simulink model "sampleModel1578"  (R2023a)
settings: Solver=VariableStepAuto  StartTime=0.0  StopTime=10.0  RelTol=1e-3
libraries: hdlsllib x5, simulink x4
settings Model: Creator=user1  LastModifiedBy=user1

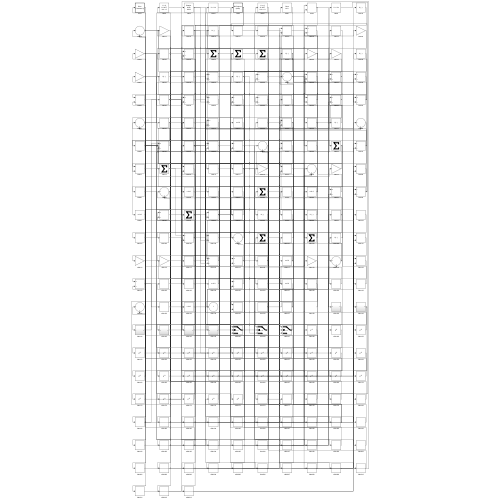
[thumbnail: Simulink's stored preview of the top-level diagram]
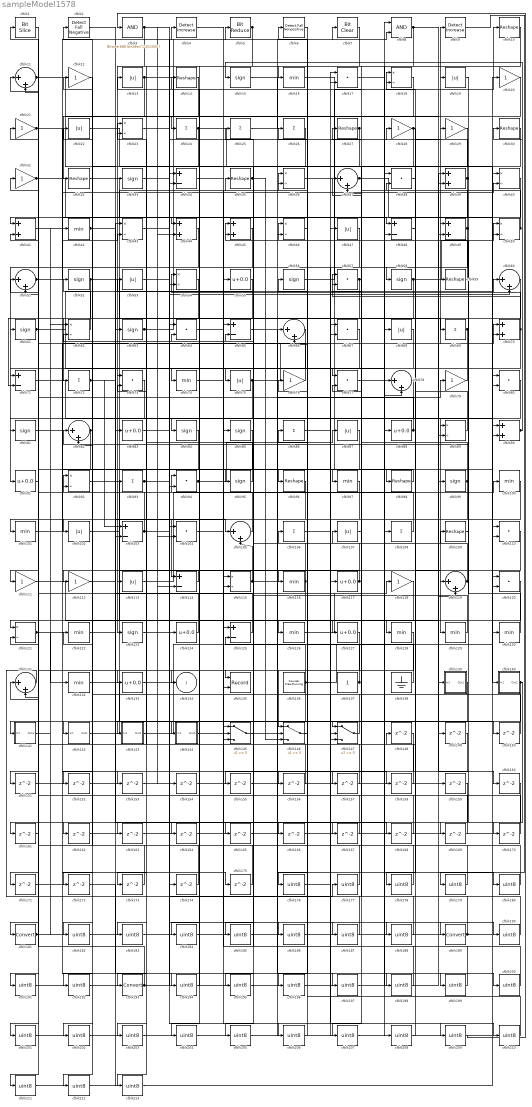
== system sampleModel1578 ==
  cfblk1 : hdlsllib/Logic and Bit Operations/Bit Slice  lidx=7  ridx=0
  cfblk{10,14,27,30,32,35,59,96,98,109} (10 alike) : Reshape
  cfblk{16,42,74,97,100..101,116,122,126,128..130,132} (13 alike) : MinMax
  cfblk{13,19,22,47,53,68,75,87,102,107,113} (11 alike) : Abs  SaturateOnIntegerOverflow=off
  cfblk{34,48,65,71,103,114,125} (7 alike) : Sum  Inputs=+-
  cfblk{17,38,57,64,67,73,77,80,94,104,110,120} (12 alike) : DotProduct  OutDataTypeStr=Inherit: Inherit via internal rule
  cfblk{11,37,51,60,66,78,82,105,119,131} (10 alike) : Sum  Inputs=|++
  cfblk{24..26,69,72,86,93,106,108} (9 alike) : Sum  Inputs=+
  cfblk{12,20..21,28..29,31,76,79,111..112,118} (11 alike) : Gain
  cfblk{18,23,36,40,43,46,50,54,62,89,92,115,121} (13 alike) : Product  Inputs=*/  RndMeth=Zero  SaturateOnIntegerOverflow=on
  cfblk{55,83,88,91,117,124,127,133} (8 alike) : Bias  Bias=0.0  SaturateOnIntegerOverflow=off
  cfblk{15,33,52,56,58,61,63,81,84..85,95,99,123} (13 alike) : Signum
  cfblk135 : Record  FileSettingsInternal="{\"entries\":[{\"content\":{\"excelSettings\":{\"content\":{},\"type\":\"Streamout.ExcelSettings\"}},\"type\":\"Streamout.FileSettingStorage\",\"uuid\":\"\"}],\"packageUris\":[\"http:\\/\\/schema.mathworks.com\\/mf0\\/streamout_blocks\\/R2020a\"],\"version\":\"1.0\"}"  Layout=[1 1]  SignalsInternal="{\"entries\":[{\"content\":{\"signals\":[{\"content\":{\"blockPath\":[],\"dimensions\":[1],\"domain\":\"\",\"lineColor\":\"#a2142f\",\"plots\":[1],\"port\":1,\"signalID\":1922,\"signalName\":\"XY Graph:1\"},\"type\":\"RecordBlkView.Signal\",\"uuid\":\"\"},{\"content\":{\"blockPath\":[],\"dimensions\":[1],\"domain\":\"\",\"lineColor\":\"#139fff\",\"plots\":[1],\"port\":2,\"signalID\":1925,\"signalName\":\"XY Graph:2\"},\"type\":\"RecordBlkView.Signal\",\"uuid\":\"\"}]},\"type\":\"RecordBlkView.InputSignals\",\"uuid\":\"\"}],\"packageUris\":[\"http:\\/\\/schema.mathworks.com\\/mf0\\/streamout_blocks\\/R2020a\"],\"version\":\"1.0\"}"  VisualizationBindings="{\"xyplotplugin\":{\"info\":[{\"series\":[{\"bindingParametersList\":[{\"parameter\":\"X-Axis\",\"signalID\":1922,\"signalName\":\"XY Graph:1\"},{\"parameter\":\"Y-Axis\",\"signalID\":1925,\"signalName\":\"XY Graph:2\"}],\"seriesID\":19021}],\"subplotID\":1}]}}"  CompatibilityTag=XY  st=-1
  cfblk136 : hdlsllib/Sources/Counter Free-Running  NumBits=16  tsamp=-1
  cfblk137 : Constant  SampleTime=-1
  cfblk138 : Ground
  cfblk139 : Subsystem
      settings: LibrarySourceBlock=|
      | hdlsllib/Ports &
      | Subsystems/Subsystem
  cfblk140 : Subsystem
      settings: LibrarySourceBlock=|
      | hdlsllib/Ports &
      | Subsystems/Subsystem
  cfblk141 : Subsystem
      settings: LibrarySourceBlock=|
      | hdlsllib/Ports &
      | Subsystems/Subsystem
  cfblk142 : Subsystem
      settings: LibrarySourceBlock=|
      | hdlsllib/Ports &
      | Subsystems/Subsystem
  cfblk143 : Subsystem
      settings: LibrarySourceBlock=|
      | hdlsllib/Ports &
      | Subsystems/Subsystem
  cfblk144 : Subsystem
      settings: LibrarySourceBlock=|
      | hdlsllib/Ports &
      | Subsystems/Subsystem
  cfblk145 : Switch  SaturateOnIntegerOverflow=off  InputSameDT=off
  cfblk146 : Switch  SaturateOnIntegerOverflow=off  InputSameDT=off
  cfblk147 : Switch  SaturateOnIntegerOverflow=off  InputSameDT=off
  cfblk{148..175} (28 alike) : Delay  SampleTime=1
  cfblk{176..180,182..188,190..192,194..213} (35 alike) : DataTypeConversion  OutDataTypeStr=uint8  SaturateOnIntegerOverflow=off  RndMeth=Floor
  cfblk181 : DataTypeConversion  SaturateOnIntegerOverflow=off  RndMeth=Floor
  cfblk189 : DataTypeConversion  SaturateOnIntegerOverflow=off  RndMeth=Floor
  cfblk193 : DataTypeConversion  SaturateOnIntegerOverflow=off  RndMeth=Floor
  cfblk2 : hdlsllib/Logic and Bit Operations/Detect Fall Negative  vinit=0  OutDataTypeStr=boolean
  cfblk3 : simulink/Logic and Bit Operations/Bitwise Operator  logicop=AND  UseBitMask=on  BitMask=bin2dec('11011001')  BitMaskRealWorld=Stored Integer
      settings: LibrarySourceBlock=|
      | hdlsllib/Logic and Bit
      | Operations/Bitwise
      | Operator
  cfblk{39,41,44..45,49,70,90} (7 alike) : Sum
  cfblk4 : simulink/Logic and Bit Operations/Detect Increase  vinit=0.0  OutDataTypeStr=boolean
      settings: LibrarySourceBlock=|
      | hdlsllib/Logic and Bit
      | Operations/Detect
      | Increase
  cfblk5 : hdlsllib/Logic and Bit Operations/Bit Reduce  mode=AND
  cfblk6 : hdlsllib/Logic and Bit Operations/Detect Fall Nonpositive  vinit=0  OutDataTypeStr=boolean
  cfblk7 : simulink/Logic and Bit Operations/Bit Clear  iBit=0
      settings: LibrarySourceBlock=|
      | hdlsllib/Logic and Bit
      | Operations/Bit Clear
  cfblk8 : Logic  AllPortsSameDT=off  OutDataTypeStr=boolean
  cfblk9 : simulink/Logic and Bit Operations/Detect Increase  vinit=0.0  OutDataTypeStr=boolean
      settings: LibrarySourceBlock=|
      | hdlsllib/Logic and Bit
      | Operations/Detect
      | Increase
  cfblk134 : Outport  VectorParamsAs1DForOutWhenUnconnected=off
  wires:
  cfblk141/1(Out1) -> cfblk42/1
  cfblk98/1 -> cfblk97/1
  cfblk63/1 -> cfblk5/1, cfblk7/1, cfblk104/2
  cfblk117/1 -> cfblk2/1, cfblk113/1
  cfblk44/1 -> cfblk91/1
  cfblk49/1 -> cfblk16/1, cfblk147/3
  cfblk108/1 -> cfblk94/1
  cfblk58/1 -> cfblk50/1, cfblk71/2
  cfblk90/1 -> cfblk15/1, cfblk30/1
  cfblk110/1 -> cfblk128/1
  cfblk59/1 -> cfblk45/1
  cfblk140/1(Out1) -> cfblk170/1, cfblk171/1
  cfblk43/1 -> cfblk124/1
  cfblk137/1 -> cfblk135/1, cfblk36/2
  cfblk56/1 -> cfblk28/1
  cfblk142/1(Out1) -> cfblk35/1
  cfblk129/1 -> cfblk45/2
  cfblk31/1 -> cfblk123/1, cfblk98/1
  cfblk32/1 -> cfblk48/1
  cfblk80/1 -> cfblk181/1
  cfblk132/1 -> cfblk147/1
  cfblk3/1 -> cfblk73/1, cfblk96/1, cfblk154/1
  cfblk18/1 -> cfblk24/1
  cfblk103/1 -> cfblk92/1, cfblk150/1
  cfblk130/1 -> cfblk82/1
  cfblk2/1 -> cfblk105/1
  cfblk40/1 -> cfblk116/1
  cfblk75/1 -> cfblk9/1, cfblk173/1, cfblk180/1
  cfblk55/1 -> cfblk61/1
  cfblk36/1 -> cfblk10/1
  cfblk69/1 -> cfblk82/2, cfblk169/1
  cfblk71/1 -> cfblk129/1
  cfblk52/1 -> cfblk121/1, cfblk94/2
  cfblk138/1 -> cfblk26/1
  cfblk14/1 -> cfblk193/1
  cfblk45/1 -> cfblk102/1
  cfblk37/1 -> cfblk140/1(In1), cfblk190/1
  cfblk144/1(Out1) -> cfblk100/1
  cfblk54/1 -> cfblk72/1
  cfblk62/1 -> cfblk52/1
  cfblk133/1 -> cfblk55/1
  cfblk143/1(Out1) -> cfblk20/1
  cfblk7/1 -> cfblk33/1
  cfblk16/1 -> cfblk130/1
  cfblk101/1 -> cfblk70/1
  cfblk61/1 -> cfblk19/1, cfblk104/1, cfblk93/1, cfblk108/1, cfblk175/1
  cfblk87/1 -> cfblk143/1(In1)
  cfblk48/1 -> cfblk18/1
  cfblk73/1 -> cfblk81/1
  cfblk124/1 -> cfblk21/1
  cfblk12/1 -> cfblk142/1(In1)
  cfblk8/1 -> cfblk48/2, cfblk160/1
  cfblk105/1 -> cfblk51/1
  cfblk82/1 -> cfblk111/1, cfblk152/1
  cfblk51/1 -> cfblk40/2, cfblk4/1
  cfblk24/1 -> cfblk68/1, cfblk192/1
  cfblk96/1 -> cfblk131/2
  cfblk29/1 -> cfblk34/2
  cfblk113/1 -> cfblk39/1
  cfblk109/1 -> cfblk49/1
  cfblk94/1 -> cfblk87/1, cfblk36/1
  cfblk72/1 -> cfblk77/1, cfblk103/1
  cfblk20/1 -> cfblk32/1
  cfblk57/1 -> cfblk166/1, cfblk167/1
  cfblk123/1 -> cfblk29/1
  cfblk22/1 -> cfblk50/2
  cfblk107/1 -> cfblk57/1
  cfblk76/1 -> cfblk11/1
  cfblk104/1 -> cfblk60/1
  cfblk122/1 -> cfblk118/1
  cfblk11/1 -> cfblk83/1, cfblk59/1
  cfblk84/1 -> cfblk101/1
  cfblk10/1 -> cfblk134/1
  cfblk111/1 -> cfblk139/1(In1)
  cfblk126/1 -> cfblk8/1
  cfblk5/1 -> cfblk163/1, cfblk203/1
  cfblk147/1 -> cfblk22/1
  cfblk35/1 -> cfblk146/3, cfblk185/1
  cfblk99/1 -> cfblk77/2, cfblk182/1
  cfblk88/1 -> cfblk84/1, cfblk51/2
  cfblk28/1 -> cfblk127/1, cfblk58/1
  cfblk102/1 -> cfblk126/1
  cfblk92/1 -> cfblk119/1
  cfblk34/1 -> cfblk115/1
  cfblk106/1 -> cfblk189/1
  cfblk79/1 -> cfblk74/1
  cfblk30/1 -> cfblk75/1
  cfblk121/1 -> cfblk132/1, cfblk200/1
  cfblk70/1 -> cfblk54/1, cfblk57/2, cfblk202/1
  cfblk50/1 -> cfblk13/1, cfblk44/1
  cfblk100/1 -> cfblk114/1
  cfblk125/1 -> cfblk23/1
  cfblk93/1 -> cfblk54/2, cfblk114/2
  cfblk41/1 -> cfblk43/2
  cfblk19/1 -> cfblk89/1
  cfblk95/1 -> cfblk73/2
  cfblk39/1 -> cfblk18/2, cfblk71/1
  cfblk83/1 -> cfblk145/3
  cfblk27/1 -> cfblk95/1, cfblk165/1
  cfblk13/1 -> cfblk125/1, cfblk44/2, cfblk162/1, cfblk213/1
  cfblk128/1 -> cfblk146/1
  cfblk114/1 -> cfblk112/1
  cfblk146/1 -> cfblk76/1
  cfblk127/1 -> cfblk141/1(In1)
  cfblk89/1 -> cfblk46/1
  cfblk21/1 -> cfblk46/2, cfblk194/1
  cfblk85/1 -> cfblk133/1
  cfblk17/1 -> cfblk90/2
  cfblk25/1 -> cfblk8/2
  cfblk116/1 -> cfblk53/1, cfblk155/1
  cfblk68/1 -> cfblk144/1(In1)
  cfblk115/1 -> cfblk79/1, cfblk105/2
  cfblk33/1 -> cfblk60/2
  cfblk1/1 -> cfblk41/1
  cfblk97/1 -> cfblk135/2
  cfblk119/1 -> cfblk109/1, cfblk37/2
  cfblk136/1 -> cfblk89/2, cfblk146/2, cfblk25/1
  cfblk42/1 -> cfblk69/1, cfblk147/2, cfblk168/1
  cfblk150/1 -> cfblk34/1
  cfblk139/1(Out1) -> cfblk151/1
  cfblk151/1 -> cfblk115/2
  cfblk152/1 -> cfblk92/2
  cfblk81/1 -> cfblk153/1
  cfblk154/1 -> cfblk119/2
  cfblk155/1 -> cfblk125/2
  cfblk53/1 -> cfblk156/1
  cfblk156/1 -> cfblk23/2
  cfblk4/1 -> cfblk157/1
  cfblk157/1 -> cfblk131/1
  cfblk112/1 -> cfblk158/1
  cfblk158/1 -> cfblk43/1
  cfblk91/1 -> cfblk161/1
  cfblk161/1 -> cfblk121/2
  cfblk162/1 -> cfblk70/2
  cfblk163/1 -> cfblk145/2
  cfblk60/1 -> cfblk164/1
  cfblk164/1 -> cfblk49/2
  cfblk165/1 -> cfblk17/2
  cfblk166/1 -> cfblk90/1
  cfblk167/1 -> cfblk11/2
  cfblk168/1 -> cfblk41/2
  cfblk169/1 -> cfblk37/1
  cfblk170/1 -> cfblk145/1
  cfblk171/1 -> cfblk103/2
  cfblk118/1 -> cfblk172/1
  cfblk173/1 -> cfblk62/2
  cfblk174/1 -> cfblk1/1
  cfblk175/1 -> cfblk12/1
  cfblk6/1 -> cfblk176/1
  cfblk176/1 -> cfblk117/1
  cfblk131/1 -> cfblk177/1
  cfblk177/1 -> cfblk6/1
  cfblk38/1 -> cfblk178/1
  cfblk178/1 -> cfblk122/1
  cfblk9/1 -> cfblk179/1
  cfblk179/1 -> cfblk38/1
  cfblk180/1 -> cfblk38/2
  cfblk181/1 -> cfblk149/1, cfblk62/1
  cfblk182/1 -> cfblk80/1
  cfblk160/1 -> cfblk183/1
  cfblk183/1 -> cfblk80/2
  cfblk47/1 -> cfblk184/1
  cfblk184/1 -> cfblk85/1
  cfblk185/1 -> cfblk47/1
  cfblk64/1 -> cfblk186/1
  cfblk186/1 -> cfblk88/1
  cfblk15/1 -> cfblk187/1
  cfblk187/1 -> cfblk64/1
  cfblk153/1 -> cfblk188/1
  cfblk188/1 -> cfblk64/2
  cfblk189/1 -> cfblk56/1, cfblk107/1, cfblk27/1
  cfblk190/1 -> cfblk106/1
  cfblk159/1 -> cfblk191/1
  cfblk191/1 -> cfblk39/2
  cfblk192/1 -> cfblk159/1
  cfblk193/1 -> cfblk174/1, cfblk31/1
  cfblk194/1 -> cfblk14/1
  cfblk78/1 -> cfblk195/1
  cfblk195/1 -> cfblk99/1
  cfblk46/1 -> cfblk196/1
  cfblk196/1 -> cfblk78/1
  cfblk145/1 -> cfblk197/1
  cfblk197/1 -> cfblk78/2
  cfblk65/1 -> cfblk198/1
  cfblk198/1 -> cfblk17/1
  cfblk172/1 -> cfblk199/1
  cfblk199/1 -> cfblk65/1
  cfblk200/1 -> cfblk65/2
  cfblk67/1 -> cfblk201/1
  cfblk201/1 -> cfblk40/1
  cfblk202/1 -> cfblk67/1
  cfblk203/1 -> cfblk67/2
  cfblk66/1 -> cfblk204/1
  cfblk204/1 -> cfblk110/2
  cfblk149/1 -> cfblk205/1
  cfblk205/1 -> cfblk66/1
  cfblk74/1 -> cfblk206/1
  cfblk206/1 -> cfblk66/2
  cfblk148/1 -> cfblk207/1
  cfblk207/1 -> cfblk110/1
  cfblk77/1 -> cfblk208/1
  cfblk208/1 -> cfblk148/1
  cfblk86/1 -> cfblk209/1
  cfblk209/1 -> cfblk3/1
  cfblk23/1 -> cfblk210/1
  cfblk210/1 -> cfblk86/1
  cfblk120/1 -> cfblk211/1
  cfblk211/1 -> cfblk63/1
  cfblk26/1 -> cfblk212/1
  cfblk212/1 -> cfblk120/1
  cfblk213/1 -> cfblk120/2

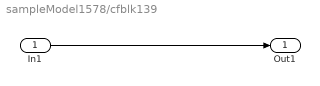
== system sampleModel1578/cfblk139 ==
  In1 : Inport
  Out1 : Outport
  wires:
  In1/1 -> Out1/1

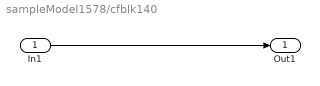
== system sampleModel1578/cfblk140 ==
  In1 : Inport
  Out1 : Outport
  wires:
  In1/1 -> Out1/1

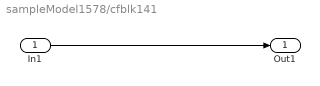
== system sampleModel1578/cfblk141 ==
  In1 : Inport
  Out1 : Outport
  wires:
  In1/1 -> Out1/1

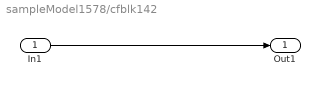
== system sampleModel1578/cfblk142 ==
  In1 : Inport
  Out1 : Outport
  wires:
  In1/1 -> Out1/1

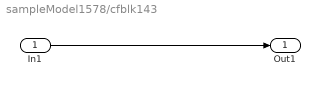
== system sampleModel1578/cfblk143 ==
  In1 : Inport
  Out1 : Outport
  wires:
  In1/1 -> Out1/1

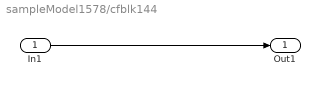
== system sampleModel1578/cfblk144 ==
  In1 : Inport
  Out1 : Outport
  wires:
  In1/1 -> Out1/1
